simulink model "power_10MW5_diode"  (R2023b)
settings: Solver=FixedStepDiscrete  StartTime=0.0  StopTime=2.6  RelTol=1e-3
InitFcn:
  | power_sysinit
StopFcn:
  | ans = [pl_T1(end),max(tem_T1),pl_T2(end),max(tem_T2),pl_D1(end),max(tem_D1),...
  |     pl_D2(end),max(tem_D2),pl_D5(end),max(tem_D5),i_45(end),i_15(end),pl_D7(end),max(tem_D7)]
values from neighbouring files (symbols this model uses):
  C_absorption = 34e-6    (= 3.4e-05)    [power_sysinit.m]
  f = 40    [power_sysinit.m]
  f_switch = 900    [power_sysinit.m]
  IN = 0.3    [power_sysinit.m]
  L_absorption = 4e-6    (= 4e-06)    [power_sysinit.m]
  m = 1/75*f    (= 0.533333333333)    [power_sysinit.m]
  PM = 0    [power_sysinit.m]
  R_absorption = 0.45    [power_sysinit.m]
  TC = 1/f_switch    (= 0.00111111111111)    [power_sysinit.m]
  temp_init = 40    [power_sysinit.m]
  Ts1 = 1e-6    (= 1e-06)    [power_sysinit.m]
  Ts2 = 500E-6    (= 0.0005)    [power_sysinit.m]
  Udc = 2500    [power_sysinit.m]
undefined symbols (not defined in the file or in its folder): DIODE_204520, DIODE_344520, DIODE_364520, DIODE_364521, DIODE_D1031SH, DIODE_D1331SH, IGCT_364520_36, IGCT_364521_36, IGCT_654522_6, magnitude, Rth_h, Rth_h_tau
libraries: spsMeanLib x138, simulink x32, spsSeriesRLCBranchLib x30, spsRMSLib x24, spsCurrentMeasurementLib x21, dspstat3 x13, spsDiodeLib x12, spsVoltageMeasurementLib x12, spsOnDelayLib x6, powerlib_extras x5, spsDCVoltageSourceLib x4, spsIGBTDiodeLib x4
(part 2 of 6)

== system power_10MW5_diode/JUNCTION LOSS and TEMP/DIODE/36L4521_D ==
  i : Inport
  PWM1 : Inport  Port=2
  PWM2 : Inport  Port=3
  PWM3 : Inport  Port=4
  PWM4 : Inport  Port=5
  U_D7 : Inport  Port=6
  I_D7 : Inport  Port=7
  36l4521_MAIN : Subsystem
  Bus Creator : BusCreator  Inputs=6
  Bus Creator1 : BusCreator  Inputs=6
  Bus Creator2 : BusCreator  Inputs=7
  Bus Creator3 : BusCreator  Inputs=3
  Bus Selector : BusSelector  OutputSignals=D1_TEMP,D1_LOSS_MEAN
  Bus Selector1 : BusSelector  OutputSignals=D2_TEMP,D2_LOSS_MEAN
  Bus Selector2 : BusSelector  OutputSignals=D5_TEMP,D5_LOSS_MEAN
  Bus Selector3 : BusSelector  OutputSignals=D7_TEMP,D7_LOSS_MEAN
  Constant{,1,3,5} (4 alike) : Constant
  Constant{2,4,6..7} (4 alike) : Constant  Value=0
  Logical Operator : Logic  Operator=OR  Inputs=4  AllPortsSameDT=off  OutDataTypeStr=boolean
  Switch{,1..3} (4 alike) : Switch  Criteria=u2 > Threshold  Threshold=DIODE_364521.Junc_temp_lim  SaturateOnIntegerOverflow=off  InputSameDT=off
  D1_BUS : Outport
  D2_BUS : Outport  Port=2
  D5_BUS : Outport  Port=3
  D7_BUS : Outport  Port=4
  <D1_TEMP> : Outport  Port=5
  <D2_TEMP> : Outport  Port=6
  <D5_TEMP> : Outport  Port=7
  <D7_TEMP> : Outport  Port=8
  <D1_LOSS_MEAN> : Outport  Port=9
  <D2_LOSS_MEAN> : Outport  Port=10
  <D5_LOSS_MEAN> : Outport  Port=11
  <D7_LOSS_MEAN> : Outport  Port=12
  TEMLIM_BOOL_D : Outport  Port=13
  wires:
  Bus Selector2/2 -> <D5_LOSS_MEAN>/1  "<D5_LOSS_MEAN>"
  Constant/1 -> Switch/1
  36l4521_MAIN/11(D2_SW_MEAN) -> Bus Creator1/5
  Bus Creator1/1 -> D2_BUS/1, [D2]  "D2_BUS"
  PWM1/1 -> 36l4521_MAIN/2(PWM1)
  [D7] -> Bus Selector3/1
  36l4521_MAIN/22(D7_LOSS) -> Bus Creator3/3
  Switch3/1 -> Logical Operator/4
  Constant1/1 -> Switch2/1
  36l4521_MAIN/12(D2_SW) -> Bus Creator1/6
  36l4521_MAIN/5(D1_SW_MEAN) -> Bus Creator/5
  36l4521_MAIN/6(D1_SW) -> Bus Creator/6
  Bus Creator2/1 -> D5_BUS/1, [D5]  "D5_BUS"
  Bus Selector3/1 -> <D7_TEMP>/1, Switch3/2  "<D7_TEMP>"
  i/1 -> 36l4521_MAIN/1(i)
  Bus Selector1/1 -> <D2_TEMP>/1, Switch1/2  "<D2_TEMP>"
  Switch1/1 -> Logical Operator/2
  Bus Selector2/1 -> <D5_TEMP>/1, Switch2/2  "<D5_TEMP>"
  Constant2/1 -> Switch2/3
  PWM4/1 -> 36l4521_MAIN/5(PWM4)
  Constant4/1 -> Switch/3
  Bus Creator/1 -> D1_BUS/1, [D1]  "D1_BUS"
  36l4521_MAIN/16(D5_AVG_MEAN) -> Bus Creator2/4
  36l4521_MAIN/21(D7_LOSS_MEAN) -> Bus Creator3/2
  Switch2/1 -> Logical Operator/3
  Bus Creator3/1 -> D7_BUS/1, [D7]  "D7_BUS"
  36l4521_MAIN/7(D2_TEMP) -> Bus Creator1/1
  [D5] -> Bus Selector2/1
  Bus Selector3/2 -> <D7_LOSS_MEAN>/1  "<D7_LOSS_MEAN>"
  36l4521_MAIN/20(D7_TEMP) -> Bus Creator3/1
  36l4521_MAIN/17(D5_AVG) -> Bus Creator2/5
  36l4521_MAIN/1(D1_TEMP) -> Bus Creator/1
  PWM2/1 -> 36l4521_MAIN/3(PWM2)
  [D1] -> Bus Selector/1
  Constant3/1 -> Switch3/1
  Constant7/1 -> Switch3/3
  Constant5/1 -> Switch1/1
  36l4521_MAIN/19(D5_SW) -> Bus Creator2/7
  Bus Selector/1 -> <D1_TEMP>/1, Switch/2  "<D1_TEMP>"
  Logical Operator/1 -> TEMLIM_BOOL_D/1
  Constant6/1 -> Switch1/3
  Bus Selector1/2 -> <D2_LOSS_MEAN>/1  "<D2_LOSS_MEAN>"
  36l4521_MAIN/13(D5_TEMP) -> Bus Creator2/1
  36l4521_MAIN/15(D5_LOSS) -> Bus Creator2/3
  Switch/1 -> Logical Operator/1
  [D2] -> Bus Selector1/1
  36l4521_MAIN/18(D5_SW_MEAN) -> Bus Creator2/6
  I_D7/1 -> 36l4521_MAIN/7(I_D7)
  Bus Selector/2 -> <D1_LOSS_MEAN>/1  "<D1_LOSS_MEAN>"
  36l4521_MAIN/8(D2_LOSS_MEAN) -> Bus Creator1/2
  36l4521_MAIN/9(D2_AVG_MEAN) -> Bus Creator1/3
  U_D7/1 -> 36l4521_MAIN/6(U_D7)
  36l4521_MAIN/10(D2_AVG) -> Bus Creator1/4
  PWM3/1 -> 36l4521_MAIN/4(PWM3)
  36l4521_MAIN/14(D5_LOSS_MEAN) -> Bus Creator2/2
  36l4521_MAIN/4(D1_AVG) -> Bus Creator/4
  36l4521_MAIN/2(D1_LOSS_MEAN) -> Bus Creator/2
  36l4521_MAIN/3(D1_AVG_MEAN) -> Bus Creator/3

== system power_10MW5_diode/JUNCTION LOSS and TEMP/DIODE/D1031SH ==
  i : Inport
  PWM1 : Inport  Port=2
  PWM2 : Inport  Port=3
  PWM3 : Inport  Port=4
  PWM4 : Inport  Port=5
  U_D7 : Inport  Port=6
  I_D7 : Inport  Port=7
  Bus Creator : BusCreator  Inputs=6
  Bus Creator1 : BusCreator  Inputs=6
  Bus Creator2 : BusCreator  Inputs=7
  Bus Creator3 : BusCreator  Inputs=3
  Bus Selector : BusSelector  OutputSignals=D1_TEMP,D1_LOSS_MEAN
  Bus Selector1 : BusSelector  OutputSignals=D2_TEMP,D2_LOSS_MEAN
  Bus Selector2 : BusSelector  OutputSignals=D5_TEMP,D5_LOSS_MEAN
  Bus Selector3 : BusSelector  OutputSignals=D7_TEMP,D7_LOSS_MEAN
  Constant{,1,3,5} (4 alike) : Constant
  Constant{2,4,6..7} (4 alike) : Constant  Value=0
  D1031SH_MAIN : Subsystem
  Logical Operator : Logic  Operator=OR  Inputs=4  AllPortsSameDT=off  OutDataTypeStr=boolean
  Switch{,1..3} (4 alike) : Switch  Criteria=u2 > Threshold  Threshold=DIODE_D1031SH.Junc_temp_lim  SaturateOnIntegerOverflow=off  InputSameDT=off
  D1_BUS : Outport
  D2_BUS : Outport  Port=2
  D5_BUS : Outport  Port=3
  D7_BUS : Outport  Port=4
  <D1_TEMP> : Outport  Port=5
  <D2_TEMP> : Outport  Port=6
  <D5_TEMP> : Outport  Port=7
  <D7_TEMP> : Outport  Port=8
  <D1_LOSS_MEAN> : Outport  Port=9
  <D2_LOSS_MEAN> : Outport  Port=10
  <D5_LOSS_MEAN> : Outport  Port=11
  <D7_LOSS_MEAN> : Outport  Port=12
  TEMLIM_BOOL_D : Outport  Port=13
  wires:
  Bus Selector2/2 -> <D5_LOSS_MEAN>/1  "<D5_LOSS_MEAN>"
  Constant/1 -> Switch/1
  D1031SH_MAIN/11(D2_SW_MEAN) -> Bus Creator1/5
  Bus Creator1/1 -> D2_BUS/1, [D2]  "D2_BUS"
  PWM1/1 -> D1031SH_MAIN/2(PWM1)
  [D7] -> Bus Selector3/1
  D1031SH_MAIN/22(D7_LOSS) -> Bus Creator3/3
  Switch3/1 -> Logical Operator/4
  Constant1/1 -> Switch2/1
  D1031SH_MAIN/12(D2_SW) -> Bus Creator1/6
  D1031SH_MAIN/5(D1_SW_MEAN) -> Bus Creator/5
  D1031SH_MAIN/6(D1_SW) -> Bus Creator/6
  Bus Creator2/1 -> D5_BUS/1, [D5]  "D5_BUS"
  Bus Selector3/1 -> <D7_TEMP>/1, Switch3/2  "<D7_TEMP>"
  i/1 -> D1031SH_MAIN/1(i)
  Bus Selector1/1 -> <D2_TEMP>/1, Switch1/2  "<D2_TEMP>"
  Switch1/1 -> Logical Operator/2
  Bus Selector2/1 -> <D5_TEMP>/1, Switch2/2  "<D5_TEMP>"
  Constant2/1 -> Switch2/3
  PWM4/1 -> D1031SH_MAIN/5(PWM4)
  Constant4/1 -> Switch/3
  Bus Creator/1 -> D1_BUS/1, [D1]  "D1_BUS"
  D1031SH_MAIN/16(D5_AVG_MEAN) -> Bus Creator2/4
  D1031SH_MAIN/21(D7_LOSS_MEAN) -> Bus Creator3/2
  Switch2/1 -> Logical Operator/3
  Bus Creator3/1 -> D7_BUS/1, [D7]  "D7_BUS"
  D1031SH_MAIN/7(D2_TEMP) -> Bus Creator1/1
  [D5] -> Bus Selector2/1
  Bus Selector3/2 -> <D7_LOSS_MEAN>/1  "<D7_LOSS_MEAN>"
  D1031SH_MAIN/20(D7_TEMP) -> Bus Creator3/1
  D1031SH_MAIN/17(D5_AVG) -> Bus Creator2/5
  D1031SH_MAIN/1(D1_TEMP) -> Bus Creator/1
  PWM2/1 -> D1031SH_MAIN/3(PWM2)
  [D1] -> Bus Selector/1
  Constant3/1 -> Switch3/1
  Constant7/1 -> Switch3/3
  Constant5/1 -> Switch1/1
  D1031SH_MAIN/19(D5_SW) -> Bus Creator2/7
  Bus Selector/1 -> <D1_TEMP>/1, Switch/2  "<D1_TEMP>"
  Logical Operator/1 -> TEMLIM_BOOL_D/1
  Constant6/1 -> Switch1/3
  Bus Selector1/2 -> <D2_LOSS_MEAN>/1  "<D2_LOSS_MEAN>"
  D1031SH_MAIN/13(D5_TEMP) -> Bus Creator2/1
  D1031SH_MAIN/15(D5_LOSS) -> Bus Creator2/3
  Switch/1 -> Logical Operator/1
  [D2] -> Bus Selector1/1
  D1031SH_MAIN/18(D5_SW_MEAN) -> Bus Creator2/6
  I_D7/1 -> D1031SH_MAIN/7(I_D7)
  Bus Selector/2 -> <D1_LOSS_MEAN>/1  "<D1_LOSS_MEAN>"
  D1031SH_MAIN/8(D2_LOSS_MEAN) -> Bus Creator1/2
  D1031SH_MAIN/9(D2_AVG_MEAN) -> Bus Creator1/3
  U_D7/1 -> D1031SH_MAIN/6(U_D7)
  D1031SH_MAIN/10(D2_AVG) -> Bus Creator1/4
  PWM3/1 -> D1031SH_MAIN/4(PWM3)
  D1031SH_MAIN/14(D5_LOSS_MEAN) -> Bus Creator2/2
  D1031SH_MAIN/4(D1_AVG) -> Bus Creator/4
  D1031SH_MAIN/2(D1_LOSS_MEAN) -> Bus Creator/2
  D1031SH_MAIN/3(D1_AVG_MEAN) -> Bus Creator/3

== system power_10MW5_diode/JUNCTION LOSS and TEMP/DIODE/D1331SH ==
  i : Inport
  PWM1 : Inport  Port=2
  PWM2 : Inport  Port=3
  PWM3 : Inport  Port=4
  PWM4 : Inport  Port=5
  U_D7 : Inport  Port=6
  I_D7 : Inport  Port=7
  Bus Creator : BusCreator  Inputs=6
  Bus Creator1 : BusCreator  Inputs=6
  Bus Creator2 : BusCreator  Inputs=7
  Bus Creator3 : BusCreator  Inputs=3
  Bus Selector : BusSelector  OutputSignals=D1_TEMP,D1_LOSS_MEAN
  Bus Selector1 : BusSelector  OutputSignals=D2_TEMP,D2_LOSS_MEAN
  Bus Selector2 : BusSelector  OutputSignals=D5_TEMP,D5_LOSS_MEAN
  Bus Selector3 : BusSelector  OutputSignals=D7_TEMP,D7_LOSS_MEAN
  Constant{,1,3,5} (4 alike) : Constant
  Constant{2,4,6..7} (4 alike) : Constant  Value=0
  D1331SH_MAIN : Subsystem
  Logical Operator : Logic  Operator=OR  Inputs=4  AllPortsSameDT=off  OutDataTypeStr=boolean
  Switch{,1..3} (4 alike) : Switch  Criteria=u2 > Threshold  Threshold=DIODE_D1331SH.Junc_temp_lim  SaturateOnIntegerOverflow=off  InputSameDT=off
  D1_BUS : Outport
  D2_BUS : Outport  Port=2
  D5_BUS : Outport  Port=3
  D7_BUS : Outport  Port=4
  <D1_TEMP> : Outport  Port=5
  <D2_TEMP> : Outport  Port=6
  <D5_TEMP> : Outport  Port=7
  <D7_TEMP> : Outport  Port=8
  <D1_LOSS_MEAN> : Outport  Port=9
  <D2_LOSS_MEAN> : Outport  Port=10
  <D5_LOSS_MEAN> : Outport  Port=11
  <D7_LOSS_MEAN> : Outport  Port=12
  TEMLIM_BOOL_D : Outport  Port=13
  wires:
  D1331SH_MAIN/3(D1_AVG_MEAN) -> Bus Creator/3
  D1331SH_MAIN/2(D1_LOSS_MEAN) -> Bus Creator/2
  D1331SH_MAIN/4(D1_AVG) -> Bus Creator/4
  D1331SH_MAIN/14(D5_LOSS_MEAN) -> Bus Creator2/2
  PWM3/1 -> D1331SH_MAIN/4(PWM3)
  D1331SH_MAIN/10(D2_AVG) -> Bus Creator1/4
  U_D7/1 -> D1331SH_MAIN/6(U_D7)
  D1331SH_MAIN/9(D2_AVG_MEAN) -> Bus Creator1/3
  D1331SH_MAIN/8(D2_LOSS_MEAN) -> Bus Creator1/2
  Bus Selector/2 -> <D1_LOSS_MEAN>/1  "<D1_LOSS_MEAN>"
  I_D7/1 -> D1331SH_MAIN/7(I_D7)
  D1331SH_MAIN/18(D5_SW_MEAN) -> Bus Creator2/6
  [D2] -> Bus Selector1/1
  Switch/1 -> Logical Operator/1
  D1331SH_MAIN/15(D5_LOSS) -> Bus Creator2/3
  D1331SH_MAIN/13(D5_TEMP) -> Bus Creator2/1
  Bus Selector1/2 -> <D2_LOSS_MEAN>/1  "<D2_LOSS_MEAN>"
  Constant6/1 -> Switch1/3
  Logical Operator/1 -> TEMLIM_BOOL_D/1
  Bus Selector/1 -> Switch/2, <D1_TEMP>/1  "<D1_TEMP>"
  D1331SH_MAIN/19(D5_SW) -> Bus Creator2/7
  Constant5/1 -> Switch1/1
  Constant7/1 -> Switch3/3
  Constant3/1 -> Switch3/1
  [D1] -> Bus Selector/1
  PWM2/1 -> D1331SH_MAIN/3(PWM2)
  D1331SH_MAIN/1(D1_TEMP) -> Bus Creator/1
  D1331SH_MAIN/17(D5_AVG) -> Bus Creator2/5
  D1331SH_MAIN/20(D7_TEMP) -> Bus Creator3/1
  Bus Selector3/2 -> <D7_LOSS_MEAN>/1  "<D7_LOSS_MEAN>"
  [D5] -> Bus Selector2/1
  D1331SH_MAIN/7(D2_TEMP) -> Bus Creator1/1
  Bus Creator3/1 -> [D7], D7_BUS/1  "D7_BUS"
  Switch2/1 -> Logical Operator/3
  D1331SH_MAIN/21(D7_LOSS_MEAN) -> Bus Creator3/2
  D1331SH_MAIN/16(D5_AVG_MEAN) -> Bus Creator2/4
  Bus Creator/1 -> [D1], D1_BUS/1  "D1_BUS"
  Constant4/1 -> Switch/3
  PWM4/1 -> D1331SH_MAIN/5(PWM4)
  Constant2/1 -> Switch2/3
  Bus Selector2/1 -> Switch2/2, <D5_TEMP>/1  "<D5_TEMP>"
  Switch1/1 -> Logical Operator/2
  Bus Selector1/1 -> Switch1/2, <D2_TEMP>/1  "<D2_TEMP>"
  i/1 -> D1331SH_MAIN/1(i)
  Bus Selector3/1 -> Switch3/2, <D7_TEMP>/1  "<D7_TEMP>"
  Bus Creator2/1 -> [D5], D5_BUS/1  "D5_BUS"
  D1331SH_MAIN/6(D1_SW) -> Bus Creator/6
  D1331SH_MAIN/5(D1_SW_MEAN) -> Bus Creator/5
  D1331SH_MAIN/12(D2_SW) -> Bus Creator1/6
  Constant1/1 -> Switch2/1
  Switch3/1 -> Logical Operator/4
  D1331SH_MAIN/22(D7_LOSS) -> Bus Creator3/3
  [D7] -> Bus Selector3/1
  PWM1/1 -> D1331SH_MAIN/2(PWM1)
  Bus Creator1/1 -> [D2], D2_BUS/1  "D2_BUS"
  D1331SH_MAIN/11(D2_SW_MEAN) -> Bus Creator1/5
  Constant/1 -> Switch/1
  Bus Selector2/2 -> <D5_LOSS_MEAN>/1  "<D5_LOSS_MEAN>"

== system power_10MW5_diode/JUNCTION LOSS and TEMP/IGCT/36L4520 ==
  i : Inport
  pwm1 : Inport  Port=2
  pwm2 : Inport  Port=3
  Bus Creator : BusCreator  Inputs=7
  Bus Creator1 : BusCreator  Inputs=7
  Bus Selector : BusSelector  OutputSignals=T1_TEMP,T1_LOSS_MEAN
  Bus Selector1 : BusSelector  OutputSignals=T2_TEMP,T2_LOSS_MEAN
  Constant : Constant
  Constant4 : Constant  Value=0
  Constant5 : Constant
  Constant6 : Constant  Value=0
  Logical Operator : Logic  Operator=OR  AllPortsSameDT=off  OutDataTypeStr=boolean
  Subsystem : Subsystem
  Switch : Switch  Criteria=u2 > Threshold  Threshold=IGCT_364520_36.Junc_temp_lim  SaturateOnIntegerOverflow=off  InputSameDT=off
  Switch1 : Switch  Criteria=u2 > Threshold  Threshold=IGCT_364520_36.Junc_temp_lim  SaturateOnIntegerOverflow=off  InputSameDT=off
  T1_BUS : Outport
  T2_BUS : Outport  Port=2
  <T1_TEMP> : Outport  Port=3
  <T2_TEMP> : Outport  Port=4
  <T1_LOSS_MEAN> : Outport  Port=5
  <T2_LOSS_MEAN> : Outport  Port=6
  TEMLIM_BOOL : Outport  Port=7
  wires:
  Subsystem/5(T1_AVG) -> Bus Creator/5  "T1_AVG"
  Subsystem/10(T2_LOSS) -> Bus Creator1/3  "T2_LOSS"
  [T2] -> Bus Selector1/1
  Subsystem/11(T2_AVG_MEAN) -> Bus Creator1/4  "T2_AVG_MEAN"
  Bus Selector1/1 -> <T2_TEMP>/1, Switch1/2  "<T2_TEMP>"
  Constant4/1 -> Switch/3
  Bus Creator1/1 -> T2_BUS/1, [T2]
  Subsystem/12(T2_AVG) -> Bus Creator1/5  "T2_AVG"
  Bus Creator/1 -> T1_BUS/1, [T1]
  Switch/1 -> Logical Operator/1
  Subsystem/13(T2_SW_MEAN) -> Bus Creator1/6  "T2_SW_MEAN"
  [T1] -> Bus Selector/1
  Subsystem/4(T1_AVG_MEAN) -> Bus Creator/4  "T1_AVG_MEAN"
  Subsystem/9(T2_LOSS_MEAN) -> Bus Creator1/2  "T2_LOSS_MEAN"
  Constant6/1 -> Switch1/3
  Constant/1 -> Switch/1
  Constant5/1 -> Switch1/1
  Bus Selector/2 -> <T1_LOSS_MEAN>/1  "<T1_LOSS_MEAN>"
  pwm2/1 -> Subsystem/3(pwm2)
  Subsystem/6(T1_SW_MEAN) -> Bus Creator/6  "T1_SW_MEAN"
  Switch1/1 -> Logical Operator/2
  Bus Selector/1 -> <T1_TEMP>/1, Switch/2  "<T1_TEMP>"
  Subsystem/7(T1_SW) -> Bus Creator/7  "T1_SW"
  Bus Selector1/2 -> <T2_LOSS_MEAN>/1  "<T2_LOSS_MEAN>"
  Subsystem/1(T1_TEMP) -> Bus Creator/1  "T1_TEMP"
  Subsystem/3(T1_LOSS) -> Bus Creator/3  "T1_LOSS"
  Subsystem/2(T1_LOSS_MEAN) -> Bus Creator/2  "T1_LOSS_MEAN"
  Subsystem/14(T2_SW) -> Bus Creator1/7  "T2_SW"
  Logical Operator/1 -> TEMLIM_BOOL/1
  Subsystem/8(T2_TEMP) -> Bus Creator1/1  "T2_TEMP"
  i/1 -> Subsystem/1(i)
  pwm1/1 -> Subsystem/2(pwm1)

== system power_10MW5_diode/JUNCTION LOSS and TEMP/IGCT/36L4521 ==
  i : Inport
  pwm1 : Inport  Port=2
  pwm2 : Inport  Port=3
  Bus Creator : BusCreator  Inputs=7
  Bus Creator1 : BusCreator  Inputs=7
  Bus Selector : BusSelector  OutputSignals=T1_TEMP,T1_LOSS_MEAN
  Bus Selector1 : BusSelector  OutputSignals=T2_TEMP,T2_LOSS_MEAN
  Constant : Constant
  Constant4 : Constant  Value=0
  Constant5 : Constant
  Constant6 : Constant  Value=0
  Logical Operator : Logic  Operator=OR  AllPortsSameDT=off  OutDataTypeStr=boolean
  Subsystem : Subsystem
  Switch : Switch  Criteria=u2 > Threshold  Threshold=IGCT_364521_36.Junc_temp_lim  SaturateOnIntegerOverflow=off  InputSameDT=off
  Switch1 : Switch  Criteria=u2 > Threshold  Threshold=IGCT_364521_36.Junc_temp_lim  SaturateOnIntegerOverflow=off  InputSameDT=off
  T1_BUS : Outport
  T2_BUS : Outport  Port=2
  <T1_TEMP> : Outport  Port=3
  <T2_TEMP> : Outport  Port=4
  <T1_LOSS_MEAN> : Outport  Port=5
  <T2_LOSS_MEAN> : Outport  Port=6
  TEMLIM_BOOL : Outport  Port=7
  wires:
  pwm1/1 -> Subsystem/2(pwm1)
  i/1 -> Subsystem/1(i)
  Subsystem/8(T2_TEMP) -> Bus Creator1/1  "T2_TEMP"
  Logical Operator/1 -> TEMLIM_BOOL/1
  Subsystem/14(T2_SW) -> Bus Creator1/7  "T2_SW"
  Subsystem/2(T1_LOSS_MEAN) -> Bus Creator/2  "T1_LOSS_MEAN"
  Subsystem/3(T1_LOSS) -> Bus Creator/3  "T1_LOSS"
  Subsystem/1(T1_TEMP) -> Bus Creator/1  "T1_TEMP"
  Bus Selector1/2 -> <T2_LOSS_MEAN>/1  "<T2_LOSS_MEAN>"
  Subsystem/7(T1_SW) -> Bus Creator/7  "T1_SW"
  Bus Selector/1 -> Switch/2, <T1_TEMP>/1  "<T1_TEMP>"
  Switch1/1 -> Logical Operator/2
  Subsystem/6(T1_SW_MEAN) -> Bus Creator/6  "T1_SW_MEAN"
  pwm2/1 -> Subsystem/3(pwm2)
  Bus Selector/2 -> <T1_LOSS_MEAN>/1  "<T1_LOSS_MEAN>"
  Constant5/1 -> Switch1/1
  Constant/1 -> Switch/1
  Constant6/1 -> Switch1/3
  Subsystem/9(T2_LOSS_MEAN) -> Bus Creator1/2  "T2_LOSS_MEAN"
  Subsystem/4(T1_AVG_MEAN) -> Bus Creator/4  "T1_AVG_MEAN"
  [T1] -> Bus Selector/1
  Subsystem/13(T2_SW_MEAN) -> Bus Creator1/6  "T2_SW_MEAN"
  Switch/1 -> Logical Operator/1
  Bus Creator/1 -> [T1], T1_BUS/1
  Subsystem/12(T2_AVG) -> Bus Creator1/5  "T2_AVG"
  Bus Creator1/1 -> [T2], T2_BUS/1
  Constant4/1 -> Switch/3
  Bus Selector1/1 -> Switch1/2, <T2_TEMP>/1  "<T2_TEMP>"
  Subsystem/11(T2_AVG_MEAN) -> Bus Creator1/4  "T2_AVG_MEAN"
  [T2] -> Bus Selector1/1
  Subsystem/10(T2_LOSS) -> Bus Creator1/3  "T2_LOSS"
  Subsystem/5(T1_AVG) -> Bus Creator/5  "T1_AVG"

== system power_10MW5_diode/JUNCTION LOSS and TEMP/IGCT/65L4522 ==
  i : Inport
  pwm1 : Inport  Port=2
  pwm2 : Inport  Port=3
  Bus Creator : BusCreator  Inputs=7
  Bus Creator1 : BusCreator  Inputs=7
  Bus Selector : BusSelector  OutputSignals=T1_TEMP,T1_LOSS_MEAN
  Bus Selector1 : BusSelector  OutputSignals=T2_TEMP,T2_LOSS_MEAN
  Constant : Constant
  Constant4 : Constant  Value=0
  Constant5 : Constant
  Constant6 : Constant  Value=0
  Logical Operator : Logic  Operator=OR  AllPortsSameDT=off  OutDataTypeStr=boolean
  Subsystem : Subsystem
  Switch : Switch  Criteria=u2 > Threshold  Threshold=IGCT_654522_6.Junc_temp_lim  SaturateOnIntegerOverflow=off  InputSameDT=off
  Switch1 : Switch  Criteria=u2 > Threshold  Threshold=IGCT_654522_6.Junc_temp_lim  SaturateOnIntegerOverflow=off  InputSameDT=off
  T1_BUS : Outport
  T2_BUS : Outport  Port=2
  <T1_TEMP> : Outport  Port=3
  <T2_TEMP> : Outport  Port=4
  <T1_LOSS_MEAN> : Outport  Port=5
  <T2_LOSS_MEAN> : Outport  Port=6
  TEMLIM_BOOL : Outport  Port=7
  wires:
  pwm1/1 -> Subsystem/2(pwm1)
  i/1 -> Subsystem/1(i)
  Subsystem/8(T2_TEMP) -> Bus Creator1/1  "T2_TEMP"
  Logical Operator/1 -> TEMLIM_BOOL/1
  Subsystem/14(T2_SW) -> Bus Creator1/7  "T2_SW"
  Subsystem/2(T1_LOSS_MEAN) -> Bus Creator/2  "T1_LOSS_MEAN"
  Subsystem/3(T1_LOSS) -> Bus Creator/3  "T1_LOSS"
  Subsystem/1(T1_TEMP) -> Bus Creator/1  "T1_TEMP"
  Bus Selector1/2 -> <T2_LOSS_MEAN>/1  "<T2_LOSS_MEAN>"
  Subsystem/7(T1_SW) -> Bus Creator/7  "T1_SW"
  Bus Selector/1 -> Switch/2, <T1_TEMP>/1  "<T1_TEMP>"
  Switch1/1 -> Logical Operator/2
  Subsystem/6(T1_SW_MEAN) -> Bus Creator/6  "T1_SW_MEAN"
  pwm2/1 -> Subsystem/3(pwm2)
  Bus Selector/2 -> <T1_LOSS_MEAN>/1  "<T1_LOSS_MEAN>"
  Constant5/1 -> Switch1/1
  Constant/1 -> Switch/1
  Constant6/1 -> Switch1/3
  Subsystem/9(T2_LOSS_MEAN) -> Bus Creator1/2  "T2_LOSS_MEAN"
  Subsystem/4(T1_AVG_MEAN) -> Bus Creator/4  "T1_AVG_MEAN"
  [T1] -> Bus Selector/1
  Subsystem/13(T2_SW_MEAN) -> Bus Creator1/6  "T2_SW_MEAN"
  Switch/1 -> Logical Operator/1
  Bus Creator/1 -> [T1], T1_BUS/1
  Subsystem/12(T2_AVG) -> Bus Creator1/5  "T2_AVG"
  Bus Creator1/1 -> [T2], T2_BUS/1
  Constant4/1 -> Switch/3
  Bus Selector1/1 -> <T2_TEMP>/1, Switch1/2  "<T2_TEMP>"
  Subsystem/11(T2_AVG_MEAN) -> Bus Creator1/4  "T2_AVG_MEAN"
  [T2] -> Bus Selector1/1
  Subsystem/10(T2_LOSS) -> Bus Creator1/3  "T2_LOSS"
  Subsystem/5(T1_AVG) -> Bus Creator/5  "T1_AVG"

== system power_10MW5_diode/Subsystem1/Regulator1/1st order delay5 ==
  x : Inport
  Kd_1 : Gain  Gain=TA/0.02
  Kd_2 : Gain  Gain=0.5
  Sum1 : Sum
  Sum4 : Sum  Inputs=+-  SampleTime=TA
  Sum6 : Sum
  Unit Delay1 : UnitDelay  SampleTime=TA  HasFrameUpgradeWarning=on
  y : Outport
  wires:
  Kd_2/1 -> y/1
  Sum1/1 -> Kd_2/1
  x/1 -> Sum4/1
  Unit Delay1/1 -> Sum1/2, Sum4/2, Sum6/2
  Sum6/1 -> Sum1/1, Unit Delay1/1
  Kd_1/1 -> Sum6/1
  Sum4/1 -> Kd_1/1

== system power_10MW5_diode/Subsystem1/Regulator1/Fis ==
  En : Inport
  Constant4 : Constant
  Data Type Conversion1 : DataTypeConversion  SaturateOnIntegerOverflow=off  RndMeth=Floor
  Gain6 : Gain  Gain=2*pi
  INT1 : Subsystem
  Ki1 : Constant  Value=0
  Switch2 : Switch  Threshold=0.5  ZeroCross=off  SaturateOnIntegerOverflow=off  InputSameDT=off
  Fis1 : Outport
  wires:
  Gain6/1 -> Fis1/1
  Constant4/1 -> Switch2/1
  INT1/1(Angle) -> Gain6/1
  Data Type Conversion1/1 -> Switch2/2
  Ki1/1 -> Switch2/3
  En/1 -> Data Type Conversion1/1
  Switch2/1 -> INT1/1(Freq)

== system power_10MW5_diode/Subsystem1/Regulator1/PWM2 ==
  Uref : Inport
  EN2 : Inport  Port=2
  Data Type Conversion1 : DataTypeConversion  SaturateOnIntegerOverflow=off  RndMeth=Floor
  Data Type Conversion2 : DataTypeConversion  SaturateOnIntegerOverflow=off  RndMeth=Floor
  L_sig6 : Constant
  Logical Operator : Logic  Operator=NOT  Inputs=1  AllPortsSameDT=off  OutDataTypeStr=boolean
  Logical Operator1 : Logic  Operator=NOT  Inputs=1  AllPortsSameDT=off  OutDataTypeStr=boolean
  Logical Operator2 : Logic  AllPortsSameDT=off  OutDataTypeStr=boolean
  Logical Operator6 : Logic  AllPortsSameDT=off  OutDataTypeStr=boolean
  Logical Operator7 : Logic  Operator=OR  AllPortsSameDT=off  OutDataTypeStr=boolean
  Mux1 : Mux
  On/Off Delay{,1,6..7} (4 alike) : powerlib_extras/Control  Blocks/On//Off Delay  type_delay=On delay  delay=2e-5  ic=0
  Relational Operator : RelationalOperator  OutDataTypeStr=boolean
  Relational Operator1 : RelationalOperator  OutDataTypeStr=boolean
  Sum4 : Sum  InputSameDT=on  SaturateOnIntegerOverflow=on  OutDataTypeStr=Inherit: Same as first input
  TCW : simulink/Sources/Repeating Sequence  rep_seq_t="[0 0.0008  0.0016]"  rep_seq_y=[1 0 1]
  P1 : Outport
  wires:
  Uref/1 -> Sum4/1, Relational Operator1/1
  Logical Operator6/1 -> Logical Operator/1, On/Off Delay/1
  Relational Operator1/1 -> Logical Operator7/2, Logical Operator6/2
  Relational Operator/1 -> Logical Operator7/1, Logical Operator6/1
  Sum4/1 -> Relational Operator/1
  L_sig6/1 -> Sum4/2
  Data Type Conversion1/1 -> P1/1
  On/Off Delay7/1 -> Mux1/4
  On/Off Delay1/1 -> Mux1/3
  On/Off Delay6/1 -> Mux1/2
  On/Off Delay/1 -> Mux1/1
  Logical Operator2/1 -> Data Type Conversion1/1
  Mux1/1 -> Logical Operator2/1
  EN2/1 -> Data Type Conversion2/1
  Logical Operator7/1 -> Logical Operator1/1, On/Off Delay6/1
  TCW/1 -> Relational Operator/2, Relational Operator1/2
  Logical Operator/1 -> On/Off Delay1/1
  Logical Operator1/1 -> On/Off Delay7/1
  Data Type Conversion2/1 -> Logical Operator2/2

== system power_10MW5_diode/Subsystem1/Regulator1/Vabc_r1 ==
  Fis : Inport
  Ur : Inport  Port=2
  Product2 : Product  InputSameDT=on  SaturateOnIntegerOverflow=on  OutDataTypeStr=Inherit: Same as first input
  Saturation1 : Saturate  UpperLimit=0.98  LowerLimit=-0.98  ZeroCross=off
  Trigonometric Function2 : Trigonometry
  Va : Outport
  wires:
  Trigonometric Function2/1 -> Product2/2
  Product2/1 -> Saturation1/1
  Ur/1 -> Product2/1
  Saturation1/1 -> Va/1
  Fis/1 -> Trigonometric Function2/1

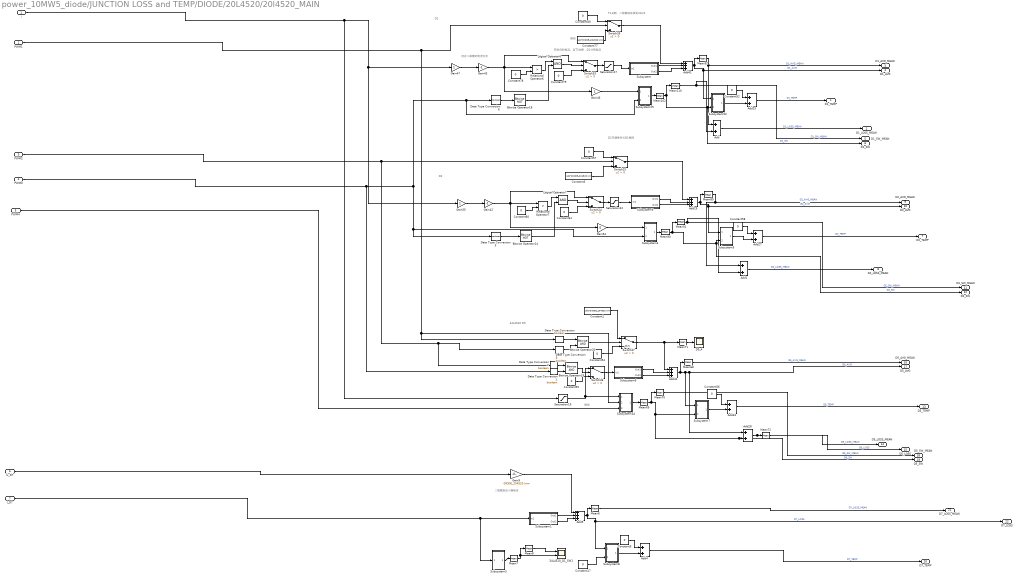
== system power_10MW5_diode/JUNCTION LOSS and TEMP/DIODE/20L4520/20l4520_MAIN ==
  note: 修改
  note: 34L4520 D5
  note: 修改
  note: 二极管反压×漏电流
  note: D2
  note: 有负向的电流、且T3关断，D1才有电流
  note: 修改
  note: 流过二极管的电流为负
  note: D2开通条件与D1相同
  note: T1关断、二极管就会承受Vdc/2
  note: D1
  i : Inport
  PWM1 : Inport  Port=2
  PWM2 : Inport  Port=3
  PWM3 : Inport  Port=4
  PWM4 : Inport  Port=5
  U_D7 : Inport  Port=6
  I_D7 : Inport  Port=7
  34L4520_D1_SW1 : Scope  NumInputPorts=2
  Add{,1,4,25,27..28,43} (7 alike) : Sum
  Add{5,29,41..42} (4 alike) : Sum  Inputs=+++
  Bitwise Operator14 : simulink/Logic and Bit Operations/Bitwise Operator  logicop=NOT  UseBitMask=off  BitMask=bin2dec('11011001')  BitMaskRealWorld=Stored Integer
  Bitwise Operator18 : simulink/Logic and Bit Operations/Bitwise Operator  logicop=NOT  UseBitMask=off  BitMask=bin2dec('11011001')  BitMaskRealWorld=Stored Integer
  Bitwise Operator19 : simulink/Logic and Bit Operations/Bitwise Operator  logicop=AND  UseBitMask=off  NumInputPorts=2  BitMask=bin2dec('11011001')  BitMaskRealWorld=Stored Integer
  Bitwise Operator20 : simulink/Logic and Bit Operations/Bitwise Operator  logicop=AND  UseBitMask=off  NumInputPorts=2  BitMask=bin2dec('11011001')  BitMaskRealWorld=Stored Integer
  Constant1 : Constant  Value=Udc*DIODE_204520.Irrm
  Constant{9,17,49,52,54..58,60..61,78..79} (13 alike) : Constant  Value=0
  Constant3 : Constant  Value=Udc*DIODE_204520.Irrm
  Constant77 : Constant  Value=Udc*DIODE_204520.Irrm
  D5_4 : Scope
  Data Type Conversion{,1..3,5..6} (6 alike) : DataTypeConversion  OutDataTypeStr=boolean  SaturateOnIntegerOverflow=off  RndMeth=Floor
  Gain42 : Gain  Gain=-1
  Gain43 : Gain  Gain=-1
  Gain46 : Gain
  Gain47 : Gain
  Gain54 : Gain  Gain=0
  Gain55 : Gain
  Gain9 : Gain  Gain=-DIODE_204520.Irrm
  Logical Operator6 : Logic  AllPortsSameDT=off  OutDataTypeStr=boolean
  Logical Operator7 : Logic  AllPortsSameDT=off  OutDataTypeStr=boolean
  Mean{7,69,90,102} (4 alike) : spsMeanLib/Mean  Freq=2000  Vinit=0  Ts=Ts1
  Mean{6,8,68,70,72,91..92,110} (8 alike) : spsMeanLib/Mean  Freq=f  Vinit=0  Ts=Ts1
  Mean71 : spsMeanLib/Mean  Freq=1  Vinit=0  Ts=Ts1
  Mean89 : spsMeanLib/Mean  Freq=f  Vinit=0  Ts=1e-6
  Relational Operator6 : RelationalOperator  Operator=>  OutDataTypeStr=boolean  RndMeth=Simplest  InputSameDT=off
  Relational Operator7 : RelationalOperator  Operator=>  OutDataTypeStr=boolean  RndMeth=Simplest  InputSameDT=off
  Saturation17 : Saturate  UpperLimit=5500  LowerLimit=0
  Saturation19 : Saturate  UpperLimit=5000  LowerLimit=0
  Saturation22 : Saturate  UpperLimit=5500  LowerLimit=0
  Subsystem : Subsystem
  Subsystem1 : Subsystem
  Subsystem29 : Subsystem
  Subsystem3 : Subsystem
  Subsystem34 : Subsystem
  Subsystem4 : Subsystem
  Subsystem5 : Subsystem
  Subsystem53 : Subsystem
  Subsystem6 : Subsystem
  Subsystem7 : Subsystem
  Subsystem8 : Subsystem
  Subsystem9 : Subsystem
  Switch{24..25,33,35..37} (6 alike) : Switch  Criteria=u2 > Threshold  SaturateOnIntegerOverflow=off  InputSameDT=off
  D1_TEMP : Outport
  D1_LOSS_MEAN : Outport  Port=2
  D1_AVG_MEAN : Outport  Port=3
  D1_AVG : Outport  Port=4
  D1_SW_MEAN : Outport  Port=5
  D1_SW : Outport  Port=6
  D2_TEMP : Outport  Port=7
  D2_LOSS_MEAN : Outport  Port=8
  D2_AVG_MEAN : Outport  Port=9
  D2_AVG : Outport  Port=10
  D2_SW_MEAN : Outport  Port=11
  D2_SW : Outport  Port=12
  D5_TEMP : Outport  Port=13
  D5_LOSS_MEAN : Outport  Port=14
  D5_LOSS : Outport  Port=15
  D5_AVG_MEAN : Outport  Port=16
  D5_AVG : Outport  Port=17
  D5_SW_MEAN : Outport  Port=18
  D5_SW : Outport  Port=19
  D7_TEMP : Outport  Port=20
  D7_LOSS_MEAN : Outport  Port=21
  D7_LOSS : Outport  Port=22
  wires:
  Add1/1 -> D2_LOSS_MEAN/1  "D2_LOSS_MEAN"
  Add/1 -> D1_LOSS_MEAN/1  "D1_LOSS_MEAN"
  Add27/1 -> D2_TEMP/1  "D2_TEMP"
  Add4/1 -> D7_TEMP/1  "D7_TEMP"
  U_D7/1 -> Gain9/1
  Mean70/1 -> D5_SW_MEAN/1  "D5_SW_MEAN"
  Subsystem/2(Out2) -> Add41/3
  Saturation17/1 -> Subsystem/1(In1)
  Constant60/1 -> Relational Operator7/2
  Gain47/1 -> Gain43/1
  Data Type Conversion6/1 -> Bitwise Operator18/1
  Constant78/1 -> Relational Operator6/2
  Data Type Conversion5/1 -> Bitwise Operator14/1
  Constant57/1 -> Switch25/1
  Bitwise Operator18/1 -> Logical Operator6/2
  Constant77/1 -> Switch35/3
  Mean89/1 -> Add1/1, D2_AVG_MEAN/1  "D2_AVG_MEAN"
  Subsystem53/1(Out1) -> Add25/2
  Constant52/1 -> Add25/1
  Add43/1 -> D5_TEMP/1  "D5_TEMP"
  Logical Operator6/1 -> Switch33/2
  Constant49/1 -> Switch35/1
  Gain46/1 -> Subsystem29/1(In1)
  Gain42/1 -> Switch24/1, Gain54/1, Relational Operator7/1
  Switch24/1 -> Saturation22/1
  Constant79/1 -> Switch33/3
  Mean92/1 -> Add/1, D1_AVG_MEAN/1  "D1_AVG_MEAN"
  Switch35/1 -> Add41/1
  Switch25/1 -> Add29/1
  Mean6/1 -> D7_LOSS_MEAN/1  "D7_LOSS_MEAN"
  Gain43/1 -> Relational Operator6/1, Gain46/1, Switch33/1
  Add41/1 -> Mean92/1, Subsystem53/1(In1), D1_AVG/1  "D1_AVG"
  Subsystem5/1(Out1) -> Add27/2
  Data Type Conversion2/1 -> Bitwise Operator19/1
  Constant55/1 -> Switch36/3
  Subsystem3/1(Out1) -> Mean7/1
  Subsystem9/2(Out2) -> Add29/3
  Switch37/1 -> Add42/1, Mean71/1
  Constant54/1 -> Switch37/3
  Subsystem7/1(Out1) -> Add43/2
  Subsystem/1(Out1) -> Add41/2
  Gain9/1 -> Add5/1
  Constant58/1 -> Add27/1
  Subsystem6/1(Out1) -> Add42/2
  Mean8/1 -> 34L4520_D1_SW1/1
  Gain54/1 -> Subsystem4/1(In1)
  Mean102/1 -> Subsystem53/2(In2), D1_SW/1, Mean110/1  "D1_SW"
  Subsystem8/1(Out1) -> Add4/2
  Subsystem4/1(Out1) -> Mean90/1
  I_D7/1 -> Subsystem1/1(In1), Subsystem3/1(In1)
  Logical Operator7/1 -> Switch24/2
  Add5/1 -> Subsystem8/1(In1), D7_LOSS/1, Mean6/1  "D7_LOSS"
  Data Type Conversion3/1 -> Bitwise Operator20/2
  Mean7/1 -> Mean8/1, 34L4520_D1_SW1/2
  Relational Operator7/1 -> Logical Operator7/1
  Constant17/1 -> Subsystem8/2(In2)
  Subsystem1/2(Out2) -> Add5/3
  Add25/1 -> D1_TEMP/1  "D1_TEMP"
  Mean69/1 -> Mean70/1, Subsystem7/2(In2), Add28/2, D5_SW/1  "D5_SW"
  Bitwise Operator20/1 -> Switch37/2
  PWM4/1 -> Subsystem34/3(In3)
  Bitwise Operator19/1 -> Switch36/2
  Mean91/1 -> Add1/2, D2_SW_MEAN/1  "D2_SW_MEAN"
  PWM2/1 -> Switch25/2, Data Type Conversion3/1, Data Type Conversion2/1
  Switch33/1 -> Saturation17/1
  Mean110/1 -> Add/2, D1_SW_MEAN/1  "D1_SW_MEAN"
  Mean71/1 -> D5_4/1
  PWM3/1 -> Subsystem4/2(In2), Data Type Conversion5/1, Subsystem29/2(In2), Data Type Conversion6/1, Data Type Conversion1/1
  i/1 -> Gain47/1, Gain55/1, Saturation19/1
  Subsystem9/1(Out1) -> Add29/2
  Data Type Conversion1/1 -> Bitwise Operator19/2
  Constant61/1 -> Switch24/3
  Mean72/1 -> D5_LOSS_MEAN/1  "D5_LOSS_MEAN"
  Mean90/1 -> Mean91/1, D2_SW/1, Subsystem5/2(In2)  "D2_SW"
  PWM1/1 -> Switch35/2, Data Type Conversion/1, Subsystem34/2(In2)
  Relational Operator6/1 -> Logical Operator6/1
  Mean68/1 -> D5_AVG_MEAN/1  "D5_AVG_MEAN"
  Saturation19/1 -> Subsystem34/1(In1), Switch36/1
  Switch36/1 -> Subsystem6/1(In1)
  Subsystem6/2(Out2) -> Add42/3
  Gain55/1 -> Gain42/1
  Constant3/1 -> Switch25/3
  Constant9/1 -> Add4/1
  Subsystem34/1(Out1) -> Mean69/1
  Add42/1 -> Mean68/1, Subsystem7/1(In1), Add28/1, D5_AVG/1  "D5_AVG"
  Data Type Conversion/1 -> Bitwise Operator20/1
  Bitwise Operator14/1 -> Logical Operator7/2
  Saturation22/1 -> Subsystem9/1(In1)
  Add29/1 -> Subsystem5/1(In1), D2_AVG/1, Mean89/1  "D2_AVG"
  Constant1/1 -> Switch37/1
  Constant56/1 -> Add43/1
  Subsystem1/1(Out1) -> Add5/2
  Subsystem29/1(Out1) -> Mean102/1
  Add28/1 -> Mean72/1, D5_LOSS/1  "D5_LOSS"

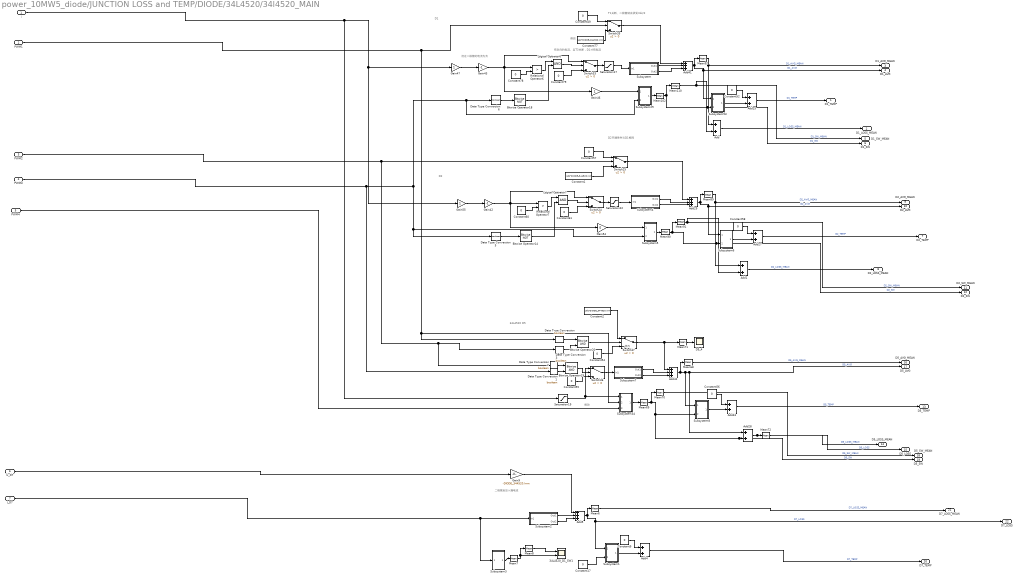
== system power_10MW5_diode/JUNCTION LOSS and TEMP/DIODE/34L4520/34l4520_MAIN ==
  note: D1
  note: T1关断、二极管就会承受Vdc/2
  note: D2开通条件与D1相同
  note: 流过二极管的电流为负
  note: 修改
  note: 有负向的电流、且T3关断，D1才有电流
  note: D2
  note: 二极管反压×漏电流
  note: 修改
  note: 34L4520 D5
  note: 修改
  i : Inport
  PWM1 : Inport  Port=2
  PWM2 : Inport  Port=3
  PWM3 : Inport  Port=4
  PWM4 : Inport  Port=5
  U_D7 : Inport  Port=6
  I_D7 : Inport  Port=7
  34L4520_D1_SW1 : Scope  NumInputPorts=2
  Add{,1,4,25,27..28,43} (7 alike) : Sum
  Add{5,29,41..42} (4 alike) : Sum  Inputs=+++
  Bitwise Operator14 : simulink/Logic and Bit Operations/Bitwise Operator  logicop=NOT  UseBitMask=off  BitMask=bin2dec('11011001')  BitMaskRealWorld=Stored Integer
  Bitwise Operator18 : simulink/Logic and Bit Operations/Bitwise Operator  logicop=NOT  UseBitMask=off  BitMask=bin2dec('11011001')  BitMaskRealWorld=Stored Integer
  Bitwise Operator19 : simulink/Logic and Bit Operations/Bitwise Operator  logicop=AND  UseBitMask=off  NumInputPorts=2  BitMask=bin2dec('11011001')  BitMaskRealWorld=Stored Integer
  Bitwise Operator20 : simulink/Logic and Bit Operations/Bitwise Operator  logicop=AND  UseBitMask=off  NumInputPorts=2  BitMask=bin2dec('11011001')  BitMaskRealWorld=Stored Integer
  Constant1 : Constant  Value=Udc*DIODE_344520.Irrm
  Constant{9,17,49,52,54..58,60..61,78..79} (13 alike) : Constant  Value=0
  Constant2 : Constant  Value=Udc*DIODE_344520.Irrm
  Constant77 : Constant  Value=Udc*DIODE_344520.Irrm
  D5_4 : Scope
  Data Type Conversion{,1..3,5..6} (6 alike) : DataTypeConversion  OutDataTypeStr=boolean  SaturateOnIntegerOverflow=off  RndMeth=Floor
  Gain42 : Gain  Gain=-1
  Gain43 : Gain  Gain=-1
  Gain46 : Gain
  Gain47 : Gain
  Gain54 : Gain  Gain=0
  Gain55 : Gain
  Gain9 : Gain  Gain=-DIODE_344520.Irrm
  Logical Operator6 : Logic  AllPortsSameDT=off  OutDataTypeStr=boolean
  Logical Operator7 : Logic  AllPortsSameDT=off  OutDataTypeStr=boolean
  Mean{7,69,90,102} (4 alike) : spsMeanLib/Mean  Freq=2000  Vinit=0  Ts=Ts1
  Mean{6,8,68,70,72,91..92,110} (8 alike) : spsMeanLib/Mean  Freq=f  Vinit=0  Ts=Ts1
  Mean71 : spsMeanLib/Mean  Freq=1  Vinit=0  Ts=Ts1
  Mean89 : spsMeanLib/Mean  Freq=f  Vinit=0  Ts=1e-6
  Relational Operator6 : RelationalOperator  Operator=>  OutDataTypeStr=boolean  RndMeth=Simplest  InputSameDT=off
  Relational Operator7 : RelationalOperator  Operator=>  OutDataTypeStr=boolean  RndMeth=Simplest  InputSameDT=off
  Saturation17 : Saturate  UpperLimit=5500  LowerLimit=0
  Saturation19 : Saturate  UpperLimit=5000  LowerLimit=0
  Saturation22 : Saturate  UpperLimit=5500  LowerLimit=0
  Subsystem : Subsystem
  Subsystem1 : Subsystem
  Subsystem2 : Subsystem
  Subsystem29 : Subsystem
  Subsystem3 : Subsystem
  Subsystem34 : Subsystem
  Subsystem4 : Subsystem
  Subsystem5 : Subsystem
  Subsystem53 : Subsystem
  Subsystem6 : Subsystem
  Subsystem7 : Subsystem
  Subsystem8 : Subsystem
  Switch{24..25,33,35..37} (6 alike) : Switch  Criteria=u2 > Threshold  SaturateOnIntegerOverflow=off  InputSameDT=off
  D1_TEMP : Outport
  D1_LOSS_MEAN : Outport  Port=2
  D1_AVG_MEAN : Outport  Port=3
  D1_AVG : Outport  Port=4
  D1_SW_MEAN : Outport  Port=5
  D1_SW : Outport  Port=6
  D2_TEMP : Outport  Port=7
  D2_LOSS_MEAN : Outport  Port=8
  D2_AVG_MEAN : Outport  Port=9
  D2_AVG : Outport  Port=10
  D2_SW_MEAN : Outport  Port=11
  D2_SW : Outport  Port=12
  D5_TEMP : Outport  Port=13
  D5_LOSS_MEAN : Outport  Port=14
  D5_LOSS : Outport  Port=15
  D5_AVG_MEAN : Outport  Port=16
  D5_AVG : Outport  Port=17
  D5_SW_MEAN : Outport  Port=18
  D5_SW : Outport  Port=19
  D7_TEMP : Outport  Port=20
  D7_LOSS_MEAN : Outport  Port=21
  D7_LOSS : Outport  Port=22
  wires:
  Add28/1 -> D5_LOSS/1, Mean72/1  "D5_LOSS"
  Subsystem29/1(Out1) -> Mean102/1
  Subsystem2/1(Out1) -> Add5/2
  Constant56/1 -> Add43/1
  Constant2/1 -> Switch37/1
  Add29/1 -> Mean89/1, D2_AVG/1, Subsystem6/1(In1)  "D2_AVG"
  Saturation22/1 -> Subsystem4/1(In1)
  Bitwise Operator14/1 -> Logical Operator7/2
  Data Type Conversion/1 -> Bitwise Operator20/1
  Add42/1 -> Subsystem8/1(In1), D5_AVG/1, Add28/1, Mean68/1  "D5_AVG"
  Subsystem34/1(Out1) -> Mean69/1
  Constant9/1 -> Add4/1
  Constant1/1 -> Switch25/3
  Gain55/1 -> Gain42/1
  Subsystem7/2(Out2) -> Add42/3
  Switch36/1 -> Subsystem7/1(In1)
  Saturation19/1 -> Switch36/1, Subsystem34/1(In1)
  Mean68/1 -> D5_AVG_MEAN/1  "D5_AVG_MEAN"
  Relational Operator6/1 -> Logical Operator6/1
  PWM1/1 -> Subsystem34/2(In2), Data Type Conversion/1, Switch35/2
  Mean90/1 -> D2_SW/1, Subsystem6/2(In2), Mean91/1  "D2_SW"
  Mean72/1 -> D5_LOSS_MEAN/1  "D5_LOSS_MEAN"
  Constant61/1 -> Switch24/3
  Data Type Conversion1/1 -> Bitwise Operator19/2
  Subsystem4/1(Out1) -> Add29/2
  i/1 -> Saturation19/1, Gain55/1, Gain47/1
  PWM3/1 -> Data Type Conversion1/1, Data Type Conversion6/1, Subsystem29/2(In2), Subsystem5/2(In2), Data Type Conversion5/1
  Mean71/1 -> D5_4/1
  Mean110/1 -> D1_SW_MEAN/1, Add/2  "D1_SW_MEAN"
  Switch33/1 -> Saturation17/1
  PWM2/1 -> Data Type Conversion2/1, Data Type Conversion3/1, Switch25/2
  Mean91/1 -> D2_SW_MEAN/1, Add1/2  "D2_SW_MEAN"
  Bitwise Operator19/1 -> Switch36/2
  PWM4/1 -> Subsystem34/3(In3)
  Bitwise Operator20/1 -> Switch37/2
  Mean69/1 -> D5_SW/1, Add28/2, Subsystem8/2(In2), Mean70/1  "D5_SW"
  Add25/1 -> D1_TEMP/1  "D1_TEMP"
  Subsystem2/2(Out2) -> Add5/3
  Constant17/1 -> Subsystem1/2(In2)
  Relational Operator7/1 -> Logical Operator7/1
  Mean7/1 -> 34L4520_D1_SW1/2, Mean8/1
  Data Type Conversion3/1 -> Bitwise Operator20/2
  Add5/1 -> Mean6/1, D7_LOSS/1, Subsystem1/1(In1)  "D7_LOSS"
  Logical Operator7/1 -> Switch24/2
  I_D7/1 -> Subsystem2/1(In1), Subsystem3/1(In1)
  Subsystem5/1(Out1) -> Mean90/1
  Subsystem1/1(Out1) -> Add4/2
  Mean102/1 -> Mean110/1, D1_SW/1, Subsystem53/2(In2)  "D1_SW"
  Gain54/1 -> Subsystem5/1(In1)
  Mean8/1 -> 34L4520_D1_SW1/1
  Subsystem7/1(Out1) -> Add42/2
  Constant58/1 -> Add27/1
  Gain9/1 -> Add5/1
  Subsystem/1(Out1) -> Add41/2
  Subsystem8/1(Out1) -> Add43/2
  Constant54/1 -> Switch37/3
  Switch37/1 -> Mean71/1, Add42/1
  Subsystem4/2(Out2) -> Add29/3
  Subsystem3/1(Out1) -> Mean7/1
  Constant55/1 -> Switch36/3
  Data Type Conversion2/1 -> Bitwise Operator19/1
  Subsystem6/1(Out1) -> Add27/2
  Add41/1 -> D1_AVG/1, Subsystem53/1(In1), Mean92/1  "D1_AVG"
  Gain43/1 -> Switch33/1, Gain46/1, Relational Operator6/1
  Mean6/1 -> D7_LOSS_MEAN/1  "D7_LOSS_MEAN"
  Switch25/1 -> Add29/1
  Switch35/1 -> Add41/1
  Mean92/1 -> D1_AVG_MEAN/1, Add/1  "D1_AVG_MEAN"
  Constant79/1 -> Switch33/3
  Switch24/1 -> Saturation22/1
  Gain42/1 -> Relational Operator7/1, Gain54/1, Switch24/1
  Gain46/1 -> Subsystem29/1(In1)
  Constant49/1 -> Switch35/1
  Logical Operator6/1 -> Switch33/2
  Add43/1 -> D5_TEMP/1  "D5_TEMP"
  Constant52/1 -> Add25/1
  Subsystem53/1(Out1) -> Add25/2
  Mean89/1 -> D2_AVG_MEAN/1, Add1/1  "D2_AVG_MEAN"
  Constant77/1 -> Switch35/3
  Bitwise Operator18/1 -> Logical Operator6/2
  Constant57/1 -> Switch25/1
  Data Type Conversion5/1 -> Bitwise Operator14/1
  Constant78/1 -> Relational Operator6/2
  Data Type Conversion6/1 -> Bitwise Operator18/1
  Gain47/1 -> Gain43/1
  Constant60/1 -> Relational Operator7/2
  Saturation17/1 -> Subsystem/1(In1)
  Subsystem/2(Out2) -> Add41/3
  Mean70/1 -> D5_SW_MEAN/1  "D5_SW_MEAN"
  U_D7/1 -> Gain9/1
  Add4/1 -> D7_TEMP/1  "D7_TEMP"
  Add27/1 -> D2_TEMP/1  "D2_TEMP"
  Add/1 -> D1_LOSS_MEAN/1  "D1_LOSS_MEAN"
  Add1/1 -> D2_LOSS_MEAN/1  "D2_LOSS_MEAN"

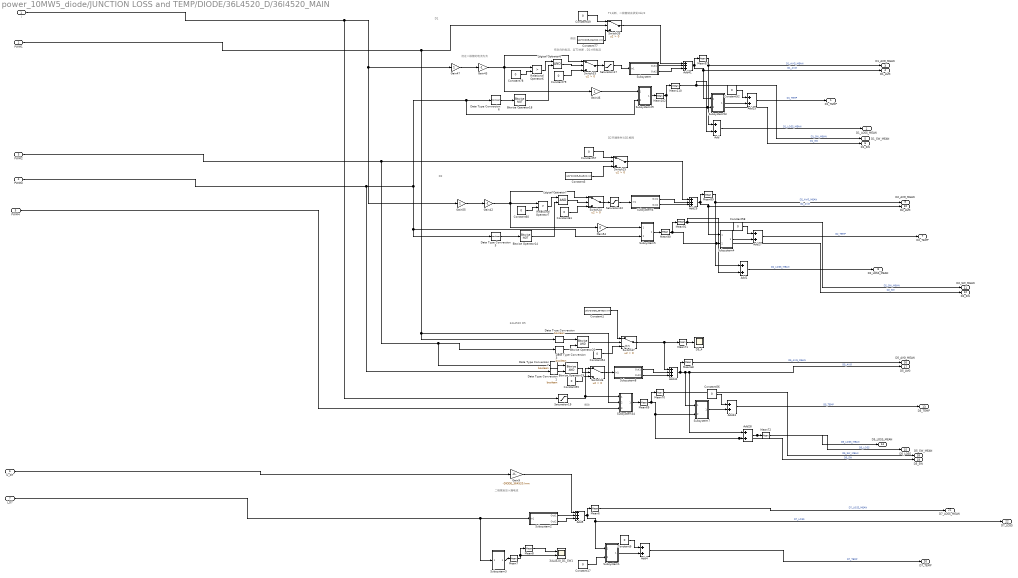
== system power_10MW5_diode/JUNCTION LOSS and TEMP/DIODE/36L4520_D/36l4520_MAIN ==
  note: 修改
  note: 34L4520 D5
  note: 修改
  note: 二极管反压×漏电流
  note: D2
  note: 有负向的电流、且T3关断，D1才有电流
  note: 修改
  note: 流过二极管的电流为负
  note: D2开通条件与D1相同
  note: T1关断、二极管就会承受Vdc/2
  note: D1
  i : Inport
  PWM1 : Inport  Port=2
  PWM2 : Inport  Port=3
  PWM3 : Inport  Port=4
  PWM4 : Inport  Port=5
  U_D7 : Inport  Port=6
  I_D7 : Inport  Port=7
  34L4520_D1_SW1 : Scope  NumInputPorts=2
  Add{,1,4,25,27..28,43} (7 alike) : Sum
  Add{5,29,41..42} (4 alike) : Sum  Inputs=+++
  Bitwise Operator14 : simulink/Logic and Bit Operations/Bitwise Operator  logicop=NOT  UseBitMask=off  BitMask=bin2dec('11011001')  BitMaskRealWorld=Stored Integer
  Bitwise Operator18 : simulink/Logic and Bit Operations/Bitwise Operator  logicop=NOT  UseBitMask=off  BitMask=bin2dec('11011001')  BitMaskRealWorld=Stored Integer
  Bitwise Operator19 : simulink/Logic and Bit Operations/Bitwise Operator  logicop=AND  UseBitMask=off  NumInputPorts=2  BitMask=bin2dec('11011001')  BitMaskRealWorld=Stored Integer
  Bitwise Operator20 : simulink/Logic and Bit Operations/Bitwise Operator  logicop=AND  UseBitMask=off  NumInputPorts=2  BitMask=bin2dec('11011001')  BitMaskRealWorld=Stored Integer
  Constant1 : Constant  Value=Udc*DIODE_364520.Irrm
  Constant{9,17,49,52,54..58,60..61,78..79} (13 alike) : Constant  Value=0
  Constant3 : Constant  Value=Udc*DIODE_364520.Irrm
  Constant77 : Constant  Value=Udc*DIODE_364520.Irrm
  D5_4 : Scope
  Data Type Conversion{,1..3,5..6} (6 alike) : DataTypeConversion  OutDataTypeStr=boolean  SaturateOnIntegerOverflow=off  RndMeth=Floor
  Gain42 : Gain  Gain=-1
  Gain43 : Gain  Gain=-1
  Gain46 : Gain
  Gain47 : Gain
  Gain54 : Gain  Gain=0
  Gain55 : Gain
  Gain9 : Gain  Gain=-DIODE_364520.Irrm
  Logical Operator6 : Logic  AllPortsSameDT=off  OutDataTypeStr=boolean
  Logical Operator7 : Logic  AllPortsSameDT=off  OutDataTypeStr=boolean
  Mean{7,69,90,102} (4 alike) : spsMeanLib/Mean  Freq=2000  Vinit=0  Ts=Ts1
  Mean{6,8,68,70,72,91..92,110} (8 alike) : spsMeanLib/Mean  Freq=f  Vinit=0  Ts=Ts1
  Mean71 : spsMeanLib/Mean  Freq=1  Vinit=0  Ts=Ts1
  Mean89 : spsMeanLib/Mean  Freq=f  Vinit=0  Ts=1e-6
  Relational Operator6 : RelationalOperator  Operator=>  OutDataTypeStr=boolean  RndMeth=Simplest  InputSameDT=off
  Relational Operator7 : RelationalOperator  Operator=>  OutDataTypeStr=boolean  RndMeth=Simplest  InputSameDT=off
  Saturation17 : Saturate  UpperLimit=5500  LowerLimit=0
  Saturation19 : Saturate  UpperLimit=5000  LowerLimit=0
  Saturation22 : Saturate  UpperLimit=5500  LowerLimit=0
  Subsystem : Subsystem
  Subsystem1 : Subsystem
  Subsystem2 : Subsystem
  Subsystem29 : Subsystem
  Subsystem3 : Subsystem
  Subsystem34 : Subsystem
  Subsystem4 : Subsystem
  Subsystem5 : Subsystem
  Subsystem53 : Subsystem
  Subsystem6 : Subsystem
  Subsystem7 : Subsystem
  Subsystem8 : Subsystem
  Switch{24..25,33,35..37} (6 alike) : Switch  Criteria=u2 > Threshold  SaturateOnIntegerOverflow=off  InputSameDT=off
  D1_TEMP : Outport
  D1_LOSS_MEAN : Outport  Port=2
  D1_AVG_MEAN : Outport  Port=3
  D1_AVG : Outport  Port=4
  D1_SW_MEAN : Outport  Port=5
  D1_SW : Outport  Port=6
  D2_TEMP : Outport  Port=7
  D2_LOSS_MEAN : Outport  Port=8
  D2_AVG_MEAN : Outport  Port=9
  D2_AVG : Outport  Port=10
  D2_SW_MEAN : Outport  Port=11
  D2_SW : Outport  Port=12
  D5_TEMP : Outport  Port=13
  D5_LOSS_MEAN : Outport  Port=14
  D5_LOSS : Outport  Port=15
  D5_AVG_MEAN : Outport  Port=16
  D5_AVG : Outport  Port=17
  D5_SW_MEAN : Outport  Port=18
  D5_SW : Outport  Port=19
  D7_TEMP : Outport  Port=20
  D7_LOSS_MEAN : Outport  Port=21
  D7_LOSS : Outport  Port=22
  wires:
  Add1/1 -> D2_LOSS_MEAN/1  "D2_LOSS_MEAN"
  Add/1 -> D1_LOSS_MEAN/1  "D1_LOSS_MEAN"
  Add27/1 -> D2_TEMP/1  "D2_TEMP"
  Add4/1 -> D7_TEMP/1  "D7_TEMP"
  U_D7/1 -> Gain9/1
  Mean70/1 -> D5_SW_MEAN/1  "D5_SW_MEAN"
  Subsystem/2(Out2) -> Add41/3
  Saturation17/1 -> Subsystem/1(In1)
  Constant60/1 -> Relational Operator7/2
  Gain47/1 -> Gain43/1
  Data Type Conversion6/1 -> Bitwise Operator18/1
  Constant78/1 -> Relational Operator6/2
  Data Type Conversion5/1 -> Bitwise Operator14/1
  Constant57/1 -> Switch25/1
  Bitwise Operator18/1 -> Logical Operator6/2
  Constant77/1 -> Switch35/3
  Mean89/1 -> Add1/1, D2_AVG_MEAN/1  "D2_AVG_MEAN"
  Subsystem53/1(Out1) -> Add25/2
  Constant52/1 -> Add25/1
  Add43/1 -> D5_TEMP/1  "D5_TEMP"
  Logical Operator6/1 -> Switch33/2
  Constant49/1 -> Switch35/1
  Gain46/1 -> Subsystem29/1(In1)
  Gain42/1 -> Switch24/1, Gain54/1, Relational Operator7/1
  Switch24/1 -> Saturation22/1
  Constant79/1 -> Switch33/3
  Mean92/1 -> Add/1, D1_AVG_MEAN/1  "D1_AVG_MEAN"
  Switch35/1 -> Add41/1
  Switch25/1 -> Add29/1
  Mean6/1 -> D7_LOSS_MEAN/1  "D7_LOSS_MEAN"
  Gain43/1 -> Relational Operator6/1, Gain46/1, Switch33/1
  Add41/1 -> Mean92/1, Subsystem53/1(In1), D1_AVG/1  "D1_AVG"
  Subsystem4/1(Out1) -> Add27/2
  Data Type Conversion2/1 -> Bitwise Operator19/1
  Constant55/1 -> Switch36/3
  Subsystem3/1(Out1) -> Mean7/1
  Subsystem6/2(Out2) -> Add29/3
  Switch37/1 -> Add42/1, Mean71/1
  Constant54/1 -> Switch37/3
  Subsystem7/1(Out1) -> Add43/2
  Subsystem/1(Out1) -> Add41/2
  Gain9/1 -> Add5/1
  Constant58/1 -> Add27/1
  Subsystem8/1(Out1) -> Add42/2
  Mean8/1 -> 34L4520_D1_SW1/1
  Gain54/1 -> Subsystem5/1(In1)
  Mean102/1 -> Subsystem53/2(In2), D1_SW/1, Mean110/1  "D1_SW"
  Subsystem1/1(Out1) -> Add4/2
  Subsystem5/1(Out1) -> Mean90/1
  I_D7/1 -> Subsystem2/1(In1), Subsystem3/1(In1)
  Logical Operator7/1 -> Switch24/2
  Add5/1 -> Subsystem1/1(In1), D7_LOSS/1, Mean6/1  "D7_LOSS"
  Data Type Conversion3/1 -> Bitwise Operator20/2
  Mean7/1 -> Mean8/1, 34L4520_D1_SW1/2
  Relational Operator7/1 -> Logical Operator7/1
  Constant17/1 -> Subsystem1/2(In2)
  Subsystem2/2(Out2) -> Add5/3
  Add25/1 -> D1_TEMP/1  "D1_TEMP"
  Mean69/1 -> Mean70/1, Subsystem7/2(In2), Add28/2, D5_SW/1  "D5_SW"
  Bitwise Operator20/1 -> Switch37/2
  PWM4/1 -> Subsystem34/3(In3)
  Bitwise Operator19/1 -> Switch36/2
  Mean91/1 -> Add1/2, D2_SW_MEAN/1  "D2_SW_MEAN"
  PWM2/1 -> Switch25/2, Data Type Conversion3/1, Data Type Conversion2/1
  Switch33/1 -> Saturation17/1
  Mean110/1 -> Add/2, D1_SW_MEAN/1  "D1_SW_MEAN"
  Mean71/1 -> D5_4/1
  PWM3/1 -> Subsystem5/2(In2), Data Type Conversion5/1, Subsystem29/2(In2), Data Type Conversion6/1, Data Type Conversion1/1
  i/1 -> Gain47/1, Gain55/1, Saturation19/1
  Subsystem6/1(Out1) -> Add29/2
  Data Type Conversion1/1 -> Bitwise Operator19/2
  Constant61/1 -> Switch24/3
  Mean72/1 -> D5_LOSS_MEAN/1  "D5_LOSS_MEAN"
  Mean90/1 -> Mean91/1, D2_SW/1, Subsystem4/2(In2)  "D2_SW"
  PWM1/1 -> Switch35/2, Data Type Conversion/1, Subsystem34/2(In2)
  Relational Operator6/1 -> Logical Operator6/1
  Mean68/1 -> D5_AVG_MEAN/1  "D5_AVG_MEAN"
  Saturation19/1 -> Subsystem34/1(In1), Switch36/1
  Switch36/1 -> Subsystem8/1(In1)
  Subsystem8/2(Out2) -> Add42/3
  Gain55/1 -> Gain42/1
  Constant3/1 -> Switch25/3
  Constant9/1 -> Add4/1
  Subsystem34/1(Out1) -> Mean69/1
  Add42/1 -> Mean68/1, Subsystem7/1(In1), Add28/1, D5_AVG/1  "D5_AVG"
  Data Type Conversion/1 -> Bitwise Operator20/1
  Bitwise Operator14/1 -> Logical Operator7/2
  Saturation22/1 -> Subsystem6/1(In1)
  Add29/1 -> Subsystem4/1(In1), D2_AVG/1, Mean89/1  "D2_AVG"
  Constant1/1 -> Switch37/1
  Constant56/1 -> Add43/1
  Subsystem2/1(Out1) -> Add5/2
  Subsystem29/1(Out1) -> Mean102/1
  Add28/1 -> Mean72/1, D5_LOSS/1  "D5_LOSS"
